simulink model "resolveCOM_th"  (R2018b)
settings: Solver=VariableStepAuto  StartTime=0.0  StopTime=0  RelTol=1e-3
undefined symbols (not defined in the file or in its folder): getVal, Rec, SDTV
libraries: dotFinder_ul x4, rayTrace_ul x4, visionconversions x3, visionsources x3, resolveCOM_ul x1
settings Model: Creator=mcobb  LastModifiedBy=mcobb

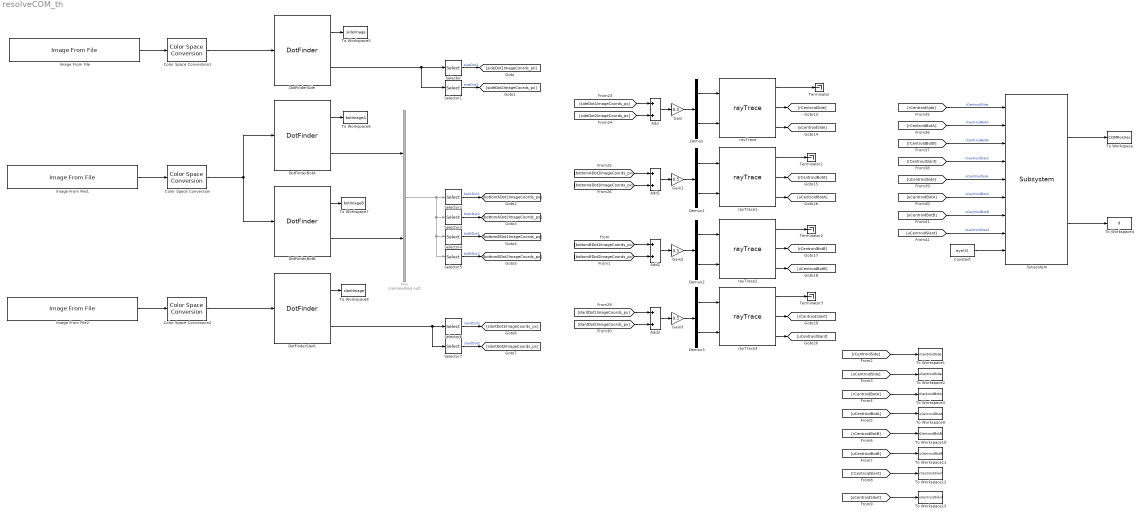
== system resolveCOM_th ==
  Add{,1..3} (4 alike) : Sum
  Color Space Conversion : visionconversions/Color Space  Conversion  conversion=Obsolete  conversionActive=R'G'B' to intensity  wp_str=D65  rec=Rec. 601 (SDTV)  sys=1125/60/2:1  imagePorts=One multidimensional signal
      settings: SourceProductName=Computer Vision System Toolbox
  Color Space Conversion1 : visionconversions/Color Space  Conversion  conversion=Obsolete  conversionActive=R'G'B' to intensity  wp_str=D65  rec=Rec. 601 (SDTV)  sys=1125/60/2:1  imagePorts=One multidimensional signal
      settings: SourceProductName=Computer Vision System Toolbox
  Color Space Conversion2 : visionconversions/Color Space  Conversion  conversion=Obsolete  conversionActive=R'G'B' to intensity  wp_str=D65  rec=Rec. 601 (SDTV)  sys=1125/60/2:1  imagePorts=One multidimensional signal
      settings: SourceProductName=Computer Vision System Toolbox
  Constant : Constant  Value=eye(3)
  Demux{,1..3} (4 alike) : Demux  Outputs=2
  DotFinderBotA : dotFinder_ul/DotFinder  ROIPositionHoldEnable=on  ROIPositionHoldCoordinates=[470 525]  ROIDimVec_px=[90 135]  ROIHalfDimVec_px=[45 67]  ROISplitDims_px=[1 45 ; 1 135 ; 46 44 ; 1 135]  DotOrientation=Vertical  OverlayOutput=on  ImageDimensions=[796 1487]  CrosshairPixelWidth_px=getVal('slntCrsHrWdth_px')
  DotFinderBotB : dotFinder_ul/DotFinder  ROIPositionHoldEnable=on  ROIPositionHoldCoordinates=[375 550]  ROIDimVec_px=[40 100]  ROIHalfDimVec_px=[20 50]  ROISplitDims_px=[1 40 ; 1 50 ; 1 40 ; 51 49]  DotOrientation=Horizontal  OverlayOutput=on  ImageDimensions=[796 1487]  CrosshairPixelWidth_px=getVal('slntCrsHrWdth_px')
  DotFinderSide : dotFinder_ul/DotFinder  ROIPositionHoldEnable=on  ROIPositionHoldCoordinates=[225 870]  ROIDimVec_px=[90 100]  ROIHalfDimVec_px=[45 50]  ROISplitDims_px=[1 90 ; 1 50 ; 1 90 ; 51 49]  DotOrientation=Horizontal  OverlayOutput=on  ImageDimensions=[796 1512]  CrosshairPixelWidth_px=getVal('slntCrsHrWdth_px')
  DotFinderSlant : dotFinder_ul/DotFinder  ROIPositionHoldEnable=on  ROIPositionHoldCoordinates=[500 620]  ROIDimVec_px=[50 100]  ROIHalfDimVec_px=[25 50]  ROISplitDims_px=[1 50 ; 1 50 ; 1 50 ; 51 49]  DotOrientation=Horizontal  OverlayOutput=on  ImageDimensions=[797 1506]  CrosshairPixelWidth_px=getVal('slntCrsHrWdth_px')
  Gain{,1..3} (4 alike) : Gain  Gain=0.5
  Image From File : visionsources/Image From File  Tag=vipblks_nd  FileName=targetScreen_Machine3_Side_Cropped.png  imagePorts=One multidimensional signal  Ts=inf  ImageDataType=Inherit from input image  Signed=on  WordLength=16  sdImageDataType=uint(8)  FractionLengthMode=User-defined  FractionLength=15  OutPortLabels=R|G|B
      settings: SourceProductName=Computer Vision System Toolbox
  Image From File1 : visionsources/Image From File  Tag=vipblks_nd  FileName=targetScreen_Machine4_Bottom_Cropped.png  imagePorts=One multidimensional signal  Ts=inf  ImageDataType=Inherit from input image  Signed=on  WordLength=16  sdImageDataType=uint(8)  FractionLengthMode=User-defined  FractionLength=15  OutPortLabels=R|G|B
      settings: SourceProductName=Computer Vision System Toolbox
  Image From File2 : visionsources/Image From File  Tag=vipblks_nd  FileName=targetScreen_Machine5_Slant_Cropped.png  imagePorts=One multidimensional signal  Ts=inf  ImageDataType=Inherit from input image  Signed=on  WordLength=16  sdImageDataType=uint(8)  FractionLengthMode=User-defined  FractionLength=15  OutPortLabels=R|G|B
      settings: SourceProductName=Computer Vision System Toolbox
  Mux : Mux  Commented=on  Inputs=2
  Selector : Selector  InputPortWidth=4  IndexOptions=Index vector (dialog)  Indices=[1 2]  OutputSizes=1
  Selector1 : Selector  InputPortWidth=4  IndexOptions=Index vector (dialog)  Indices=[3 4]  OutputSizes=1
  Selector2 : Selector  InputPortWidth=8  IndexOptions=Index vector (dialog)  Indices=[1 2]  OutputSizes=1
  Selector3 : Selector  InputPortWidth=8  IndexOptions=Index vector (dialog)  Indices=[3 4]  OutputSizes=1
  Selector4 : Selector  InputPortWidth=8  IndexOptions=Index vector (dialog)  Indices=[5 6]  OutputSizes=1
  Selector5 : Selector  InputPortWidth=8  IndexOptions=Index vector (dialog)  Indices=[7 8]  OutputSizes=1
  Selector6 : Selector  InputPortWidth=4  IndexOptions=Index vector (dialog)  Indices=[1 2]  OutputSizes=1
  Selector7 : Selector  InputPortWidth=4  IndexOptions=Index vector (dialog)  Indices=[3 4]  OutputSizes=1
  Subsystem : resolveCOM_ul/Subsystem  sideDotPosVec_cm=[0.091 4.54 0.878]  botADotPosVec_cm=[2.48 0 -4.53]  botBDotPosVec_cm=[-1 0 -4.64]
  Terminator{,1..3} (4 alike) : Terminator
  To Workspace : ToWorkspace  VariableName=COMPosVec  SaveFormat=Timeseries  SampleTime=-1
  To Workspace1 : ToWorkspace  VariableName=rCentroidSide  SaveFormat=Timeseries  SampleTime=-1
  To Workspace10 : ToWorkspace  VariableName=rCentroidBotB  SaveFormat=Timeseries  SampleTime=-1
  To Workspace11 : ToWorkspace  VariableName=uCentroidBotB  SaveFormat=Timeseries  SampleTime=-1
  To Workspace12 : ToWorkspace  VariableName=rCentroidSlant  SaveFormat=Timeseries  SampleTime=-1
  To Workspace13 : ToWorkspace  VariableName=uCentroidSlant  SaveFormat=Timeseries  SampleTime=-1
  To Workspace2 : ToWorkspace  VariableName=uCentroidSide  SaveFormat=Timeseries  SampleTime=-1
  To Workspace3 : ToWorkspace  VariableName=rCentroidBotA  SaveFormat=Timeseries  SampleTime=-1
  To Workspace4 : ToWorkspace  VariableName=d  SaveFormat=Timeseries  SampleTime=-1
  To Workspace5 : ToWorkspace  VariableName=sideImage  SampleTime=-1
  To Workspace6 : ToWorkspace  VariableName=botImageA  SampleTime=-1
  To Workspace7 : ToWorkspace  VariableName=botImageB  SampleTime=-1
  To Workspace8 : ToWorkspace  VariableName=slantImage  SampleTime=-1
  To Workspace9 : ToWorkspace  VariableName=uCentroidBotA  SaveFormat=Timeseries  SampleTime=-1
  rayTrace : rayTrace_ul/rayTrace  camPosVec_cm=getVal('sideCamPosVec_cm')  camEulAngles_deg=[0 90 90]  dist2Glass_cm=1  indOfRefVec=[1.000293,1.52,1.333]  glassPlane=2  glassThickness_cm=2  imageDimsVec_px=[796 1512]  camFOV_deg=getVal('cameraFOV_deg')
  rayTrace1 : rayTrace_ul/rayTrace  camPosVec_cm=getVal('botCamPosVec_cm')  camEulAngles_deg=[0 180 180]  dist2Glass_cm=5  indOfRefVec=[1.000293,1.52,1.333]  glassPlane=1  glassThickness_cm=2  imageDimsVec_px=[796 1487]  camFOV_deg=getVal('cameraFOV_deg')
  rayTrace2 : rayTrace_ul/rayTrace  camPosVec_cm=getVal('botCamPosVec_cm')  camEulAngles_deg=[0 180 180]  dist2Glass_cm=5  indOfRefVec=[1.000293,1.52,1.333]  glassPlane=1  glassThickness_cm=2  imageDimsVec_px=[796 1487]  camFOV_deg=getVal('cameraFOV_deg')
  rayTrace3 : rayTrace_ul/rayTrace  camPosVec_cm=getVal('slntCamPosVec_cm')  camEulAngles_deg=[0 135 180]  dist2Glass_cm=7  indOfRefVec=[1.000293,1.52,1.333]  glassPlane=1  glassThickness_cm=2  imageDimsVec_px=[797 1506]  camFOV_deg=getVal('cameraFOV_deg')
  wires:
  Demux3/2 -> rayTrace3/2
  [slantDot2ImageCoords_px] -> Add3/2
  Add1/1 -> Gain1/1
  Add3/1 -> Gain3/1
  rayTrace3/1 -> Terminator3/1
  Demux2/2 -> rayTrace2/2
  rayTrace2/1 -> Terminator2/1
  rayTrace/1 -> Terminator/1
  Demux1/2 -> rayTrace1/2
  rayTrace1/2 -> [rCentroidBotA]
  Demux3/1 -> rayTrace3/1
  [bottomADot2ImageCoords_px] -> Add1/2
  Demux/1 -> rayTrace/1
  Gain2/1 -> Demux2/1
  rayTrace2/3 -> [uCentroidBotB]
  Demux/2 -> rayTrace/2
  Demux1/1 -> rayTrace1/1
  Demux2/1 -> rayTrace2/1
  Gain1/1 -> Demux1/1
  rayTrace1/1 -> Terminator1/1
  rayTrace3/2 -> [rCentroidSlant]
  [sideDot2ImageCoords_px] -> Add/2
  Gain/1 -> Demux/1
  rayTrace1/3 -> [uCentroidBotA]
  Gain3/1 -> Demux3/1
  rayTrace2/2 -> [rCentroidBotB]
  [bottomADot1ImageCoords_px] -> Add1/1
  Add/1 -> Gain/1
  [bottomBDot2ImageCoords_px] -> Add2/2
  [slantDot1ImageCoords_px] -> Add3/1
  [sideDot1ImageCoords_px] -> Add/1
  Add2/1 -> Gain2/1
  rayTrace/2 -> [rCentroidSide]
  rayTrace3/3 -> [uCentroidSlant]
  rayTrace/3 -> [uCentroidSide]
  [bottomBDot1ImageCoords_px] -> Add2/1
  Color Space Conversion/1 -> DotFinderBotA/1, DotFinderBotB/1
  Color Space Conversion2/1 -> DotFinderSlant/1
  Image From File2/1 -> Color Space Conversion2/1
  DotFinderBotA/1 -> To Workspace6/1
  Image From File/1 -> Color Space Conversion1/1
  Image From File1/1 -> Color Space Conversion/1
  DotFinderSlant/1 -> To Workspace8/1
  Color Space Conversion1/1 -> DotFinderSide/1
  DotFinderBotB/1 -> To Workspace7/1
  DotFinderSide/1 -> To Workspace5/1
  DotFinderSlant/2 -> Selector7/1, Selector6/1
  DotFinderBotA/2 -> Mux/1
  DotFinderBotB/2 -> Mux/2
  Mux/1 -> Selector4/1, Selector5/1, Selector3/1, Selector2/1
  DotFinderSide/2 -> Selector1/1, Selector/1
  Selector/1 -> [sideDot1ImageCoords_px]  "sideDot1"
  Selector1/1 -> [sideDot2ImageCoords_px]  "sideDot2"
  Selector2/1 -> [bottomADot1ImageCoords_px]  "botADot1"
  Selector3/1 -> [bottomADot2ImageCoords_px]  "botADot2"
  Selector4/1 -> [bottomBDot1ImageCoords_px]  "botBDot1"
  Selector5/1 -> [bottomBDot2ImageCoords_px]  "botBDot2"
  Selector6/1 -> [slantDot1ImageCoords_px]  "slantDot1"
  Selector7/1 -> [slantDot2ImageCoords_px]  "slantDot2"
  Subsystem/1 -> To Workspace/1
  [rCentroidSide] -> Subsystem/1  "rCentroidSide"
  [rCentroidBotA] -> Subsystem/2  "rCentroidBotA"
  [rCentroidBotB] -> Subsystem/3  "rCentroidBotB"
  [rCentroidSlant] -> Subsystem/4  "rCentroidSlant"
  [uCentroidSide] -> Subsystem/5  "uCentroidSide"
  [uCentroidBotA] -> Subsystem/6  "uCentroidBotA"
  [uCentroidBotB] -> Subsystem/7  "uCentroidBotB"
  Constant/1 -> Subsystem/9
  [uCentroidSlant] -> Subsystem/8  "uCentroidSlant"
  Subsystem/2 -> To Workspace4/1
  [rCentroidSide] -> To Workspace1/1
  [uCentroidSide] -> To Workspace2/1
  [rCentroidBotA] -> To Workspace3/1
  [uCentroidBotA] -> To Workspace9/1
  [rCentroidBotB] -> To Workspace10/1
  [uCentroidBotB] -> To Workspace11/1
  [rCentroidSlant] -> To Workspace12/1
  [uCentroidSlant] -> To Workspace13/1
